simulink library "ILA_CONFIGSS"  (R2013b)
settings: Solver=ode45  StartTime=0.0  StopTime=10.0  RelTol=1e-3
undefined symbols (not defined in the file or in its folder): L0, Mu
libraries: dspsigops x4, dspsigattribs x2, ILA_CONFIGSS x1, dspmtrx3 x1
settings Model: Creator=kschutz  LastModifiedBy=kschutz

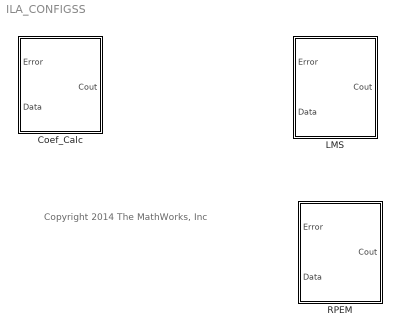
== system ILA_CONFIGSS ==
  note: Copyright 2014 The MathWorks, Inc
  Coef_Calc : Subsystem  BlockChoice=LMS
      settings: TemplateBlock=self  MemberBlocks=LMS,RPEM
  LMS : Subsystem
  RPEM : Subsystem

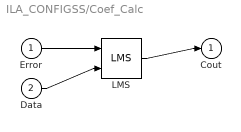
== system ILA_CONFIGSS/Coef_Calc ==
  Error : Inport
  Data : Inport  Port=2
  LMS : ILA_CONFIGSS/LMS
  Cout : Outport
  wires:
  Error/1 -> LMS/1
  Data/1 -> LMS/2
  LMS/1 -> Cout/1

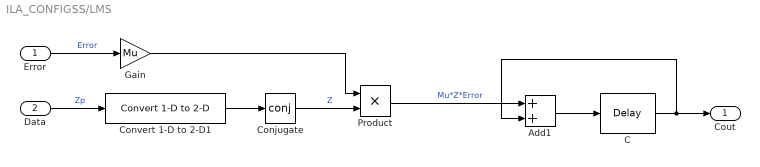
== system ILA_CONFIGSS/LMS ==
  Error : Inport
  Data : Inport  Port=2
  Add1 : Sum
  C : dspsigops/Delay  dly_unit=Samples  delay=1  ic_detail=off  dif_ic_for_ch=on  dif_ic_for_dly=off  ic=C_init  reset_popup=None
  Conjugate : Math  Operator=conj  SaturateOnIntegerOverflow=on
  Convert 1-D to 2-D1 : dspsigattribs/Convert 1-D to 2-D  M=25  N=1  frameBasedOut=off
  Gain : Gain  Gain=Mu
  Product : Product  RndMeth=Zero
  Cout : Outport
  wires:
  Gain/1 -> Product/1
  Convert 1-D to 2-D1/1 -> Conjugate/1
  Conjugate/1 -> Product/2  "Z"
  Product/1 -> Add1/1  "Mu*Z*Error"
  Error/1 -> Gain/1  "Error"
  C/1 -> Cout/1, Add1/2
  Add1/1 -> C/1
  Data/1 -> Convert 1-D to 2-D1/1  "Zp"

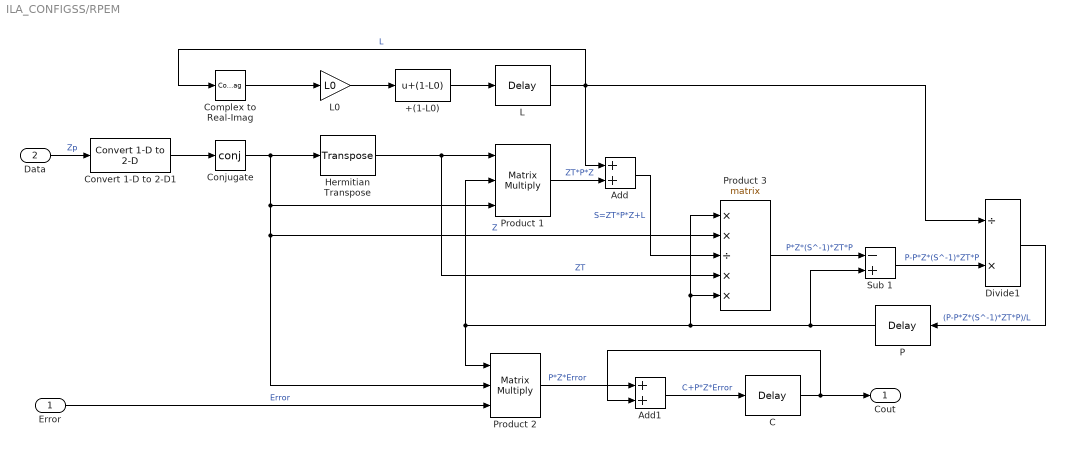
== system ILA_CONFIGSS/RPEM ==
  Error : Inport
  Data : Inport  Port=2
  +(1-L0) : Bias  Bias=(1-L0)
  Add : Sum
  Add1 : Sum
  C : dspsigops/Delay  dly_unit=Samples  delay=1  ic_detail=off  dif_ic_for_ch=on  dif_ic_for_dly=off  ic=C_init  reset_popup=None
  Complex to Real-Imag : ComplexToRealImag  Output=Real
  Conjugate : Math  Operator=conj  SaturateOnIntegerOverflow=on
  Convert 1-D to 2-D1 : dspsigattribs/Convert 1-D to 2-D  M=25  N=1  frameBasedOut=off
  Divide1 : Product  Inputs=/*
  Hermitian Transpose : dspmtrx3/Transpose  Hermitian=on  overflowFlag=off
  L : dspsigops/Delay  InputProcessing=Columns as channels (frame based)  dly_unit=Samples  delay=1  ic_detail=off  dif_ic_for_ch=off  dif_ic_for_dly=off  ic=L_init  reset_popup=None
  L0 : Gain  Gain=L0
  P : dspsigops/Delay  dly_unit=Samples  delay=1  ic_detail=off  dif_ic_for_ch=on  dif_ic_for_dly=off  ic=P0  reset_popup=None
  Product 1 : Product  Inputs=3  Multiplication=Matrix(*)
  Product 2 : Product  Inputs=3  Multiplication=Matrix(*)
  Product 3 : Product  Inputs=**/**  Multiplication=Matrix(*)
  Sub 1 : Sum  Inputs=-+
  Cout : Outport
  wires:
  Complex to Real-Imag/1 -> L0/1
  P/1 -> Sub 1/2, Product 3/1, Product 3/5, Product 1/2, Product 2/1
  L/1 -> Complex to Real-Imag/1, Divide1/1, Add/1  "L"
  Product 3/1 -> Sub 1/1  "P*Z*(S^-1)*ZT*P"
  Convert 1-D to 2-D1/1 -> Conjugate/1
  Conjugate/1 -> Product 1/3, Product 3/2, Product 2/2, Hermitian Transpose/1  "Z"
  Sub 1/1 -> Divide1/2  "P-P*Z*(S^-1)*ZT*P"
  Add/1 -> Product 3/3  "S=ZT*P*Z+L"
  Divide1/1 -> P/1  "(P-P*Z*(S^-1)*ZT*P)/L"
  Product 2/1 -> Add1/1  "P*Z*Error"
  Error/1 -> Product 2/3  "Error"
  C/1 -> Add1/2, Cout/1
  Add1/1 -> C/1  "C+P*Z*Error"
  Product 1/1 -> Add/2  "ZT*P*Z"
  Hermitian Transpose/1 -> Product 3/4, Product 1/1  "ZT"
  Data/1 -> Convert 1-D to 2-D1/1  "Zp"
  +(1-L0)/1 -> L/1
  L0/1 -> +(1-L0)/1
